simulink model "LFC_Fuzzy_AREA2"  (R2021a)
settings: Solver=VariableStepAuto  StartTime=0.0  StopTime=100  RelTol=1e-3
libraries: pid_lib x1, fuzblock x1, spspowerguiLib x1
settings Model: Creator=B.HARISH  LastModifiedBy=B.HARISH

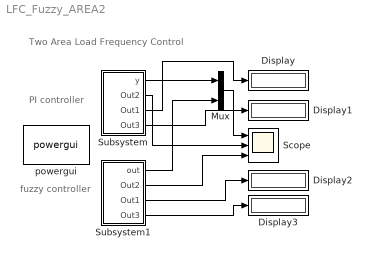
== system LFC_Fuzzy_AREA2 ==
  note: fuzzy controller
  note: PI controller
  note: Two Area Load Frequency Control
  Display{,1..3} (4 alike) : Display
  Mux : Mux  Inputs=2
  Scope : Scope  NumInputPorts=3
  Subsystem : Subsystem
  Subsystem1 : Subsystem
  powergui : spspowerguiLib/powergui  Priority=1  SimulationMode=Continuous  SampleTime=50e-6  frequency=60  Iterations=50  frequencyindice=60  Pbase=100e6  ErrMax=1e-4  UnitsV=kV  UnitsW=MW  buscounter=0  FunctionMessages=off  echomessages=off  EnableUseOfTLC=off  CurrentSourceSwitches=off  DisableSnubberDevices=off  DisableRonSwitches=off  DisableVfSwitches=off  DisplayEquations=off  AutomaticDiscreteSolvers=off  SolverType=Tustin/Backward Euler (TBE)  Interpol=off  ExternalGateDelay=off  methode=off  Ts=100  x0status=blocks  SPID=off  SwTol=0  HookPort=off  NonlinearTolerance=1e-4  nMaxIteration=100  ContinueOnMaxIteration=off  RestoreLinks=warning  ResistiveCurrentMeasurement=off  Frange=[0:2:500]  Ylog=off  Xlog=on  ShowGrid=off  save=off  variable=ZData  structure=0  ZoomFFT=off  StartTime=0.0  cycles=1  DisplayStyle=1  fundamental=60  FreqAxis=off  MaxFrequency=1000  frequencyindicesteady=1  RmsSteady=1  display=off
  wires:
  Subsystem1/2(Out2) -> Scope/3
  Subsystem/2(Out2) -> Scope/2
  Subsystem/1(y) -> Mux/1
  Subsystem1/1(out) -> Mux/2
  Mux/1 -> Scope/1
  Subsystem1/3(Out1) -> Display2/1
  Subsystem1/4(Out3) -> Display3/1
  Subsystem/3(Out1) -> Display/1
  Subsystem/4(Out3) -> Display1/1

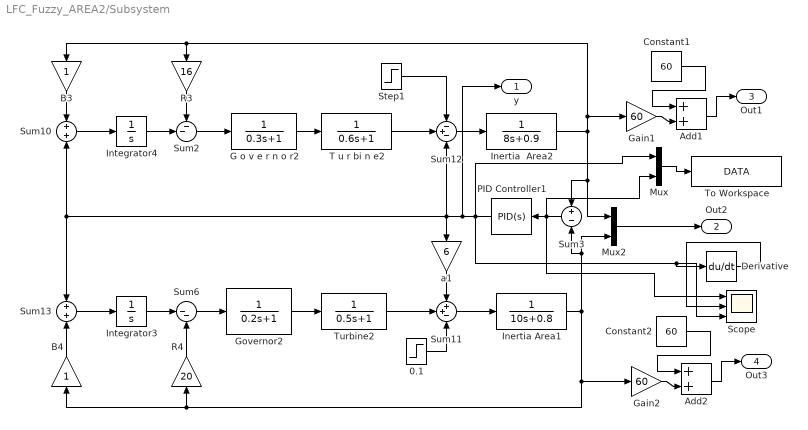
== system LFC_Fuzzy_AREA2/Subsystem ==
  0.1 : Step  Time=0  After=0.2  SampleTime=0
  Add1 : Sum
  Add2 : Sum
  B3 : Gain
  B4 : Gain
  Constant1 : Constant  Value=60
  Constant2 : Constant  Value=60
  Derivative : Derivative
  G o v e r n o r2 : TransferFcn  Denominator=[0.3 1]  ParameterTunability=Optimized
  Gain1 : Gain  Gain=60
  Gain2 : Gain  Gain=60
  Governor2 : TransferFcn  Denominator=[0.2 1]
  Inertia  Area2 : TransferFcn  Denominator=[8 0.9]
  Inertia Area1 : TransferFcn  Denominator=[10 0.8]
  Integrator3 : Integrator
  Integrator4 : Integrator
  Mux : Mux  Inputs=2
  Mux2 : Mux  Inputs=2
  PID Controller1 : pid_lib/PID Controller  Controller=PID  Form=Parallel  TimeDomain=Continuous-time  UseExternalTs=off  SampleTime=-1  IntegratorMethod=Forward Euler  FilterMethod=Forward Euler  ControllerParametersSource=internal  P=5.57550599969574  I=9.98117323449892  D=0.481439807722255  UseFilter=on  N=13.7016060269838  TunerSelectOption=Transfer Function Based (PID Tuner App)  InitialConditionSource=internal  InitialConditionForIntegrator=0  InitialConditionForFilter=0  DifferentiatorICPrevScaledInput=0  ExternalReset=none  TrackingMode=off  Kt=1  LimitOutput=off  SatLimitsSource=internal  UpperSaturationLimit=inf  LowerSaturationLimit=-inf  LinearizeAsGain=on  AntiWindupMode=none  Kb=1  POutMin=[]  POutMax=[]  IOutMin=[]  IOutMax=[]  DOutMin=[]  DOutMax=[]  NOutMin=[]  NOutMax=[]  SumOutMin=[]  SumOutMax=[]  SaturationOutMin=[]  SaturationOutMax=[]  PParamMin=[]  PParamMax=[]  IParamMin=[]  IParamMax=[]  DParamMin=[]  DParamMax=[]  NParamMin=[]  NParamMax=[]  KbParamMin=[]  KbParamMax=[]  KtParamMin=[]  KtParamMax=[]  KbOutMin=[]  KbOutMax=[]  KtOutMin=[]  KtOutMax=[]  IntegratorOutMin=[]  IntegratorOutMax=[]  FilterOutMin=[]  FilterOutMax=[]  SumI1OutMin=[]  SumI1OutMax=[]  SumI2OutMin=[]  SumI2OutMax=[]  SumI3OutMin=[]  SumI3OutMax=[]  SumI4OutMin=[]  SumI4OutMax=[]  SumDOutMin=[]  SumDOutMax=[]  DifferentiatorOutMin=[]  DifferentiatorOutMax=[]  FilterDiffOutCoefMin=[]  FilterDiffOutCoefMax=[]  ReciprocalOutMin=[]  ReciprocalOutMax=[]  SumDenOutMin=[]  SumDenOutMax=[]  SumNumOutMin=[]  SumNumOutMax=[]  DivideOutMin=[]  DivideOutMax=[]  UdiffTsProdOutMin=[]  UdiffTsProdOutMax=[]  NTsProdOutMin=[]  NTsProdOutMax=[]  UintegralTsProdOutMin=[]  UintegralTsProdOutMax=[]  UngainTsProdOutMin=[]  UngainTsProdOutMax=[]  IntegratorContinuousStateAttributes=''  IntegratorStateMustResolveToSignalObject=off  IntegratorRTWStateStorageClass=Auto  FilterContinuousStateAttributes=''  FilterStateMustResolveToSignalObject=off  FilterRTWStateStorageClass=Auto  ParallelPVariant=InternalParameters  IdealPVariant=Disabled  IVariant=InternalParameters  DVariant=InternalParameters  IntegratorVariant=Continuous  SatVariant=Disabled  AWVariant=Passthrough  PCopyVariant=Disabled  TRVariant=Disabled  FdbkBlocksVariant=Forward  IdealPFdbkVariant=Disabled  SatFdbkVariant=Disabled  DerivativeFilterVariant=ContFilter  NVariant=InternalParameters  NCopyVariant=Disabled  FilterICVariant=InternalICsFilter  IntegratorICVariant=InternalICs  ExternalResetVariant=Disabled  TRSumVariant=Passthrough  SumFdbkVariant=Disabled  SumVariant=Sum_PID  TsampFilterVariant=InternalTs  TsampNgainVariant=Passthrough  TsampIntegralVariant=Passthrough  ExternalSaturationOutDataTypeStr=Inherit: Same as second input
  R3 : Gain  Gain=16
  R4 : Gain  Gain=20
  Scope : Scope  NumInputPorts=3
  Step1 : Step  Time=0  After=0.2  SampleTime=0
  Sum10 : Sum
  Sum11 : Sum  Inputs=++-
  Sum12 : Sum  Inputs=-+-
  Sum13 : Sum
  Sum2 : Sum  Inputs=--|
  Sum3 : Sum  Inputs=+-
  Sum6 : Sum  Inputs=|--
  T u r bi n e2 : TransferFcn  Denominator=[0.6 1]
  To Workspace : ToWorkspace  VariableName=DATA  SaveFormat=Timeseries  SampleTime=-1
  Turbine2 : TransferFcn  Denominator=[0.5 1]
  a1 : Gain  Gain=6
  y : Outport
  Out2 : Outport  Port=2
  Out1 : Outport  Port=3
  Out3 : Outport  Port=4
  wires:
  PID Controller1/1 -> Derivative/1, Scope/3, y/1, a1/1, Sum13/1, Sum10/2, Sum12/3, Mux/1
  G o v e r n o r2/1 -> T u r bi n e2/1
  0.1/1 -> Sum11/3
  T u r bi n e2/1 -> Sum12/2
  a1/1 -> Sum11/1
  Inertia  Area2/1 -> Gain1/1, B3/1, R3/1, Mux2/1, Sum3/1
  Sum10/1 -> Integrator4/1
  Integrator3/1 -> Sum6/1
  R3/1 -> Sum2/1
  Sum11/1 -> Inertia Area1/1
  Sum13/1 -> Integrator3/1
  Sum6/1 -> Governor2/1
  Sum12/1 -> Inertia  Area2/1
  Turbine2/1 -> Sum11/2
  Governor2/1 -> Turbine2/1
  B4/1 -> Sum13/2
  Integrator4/1 -> Sum2/2
  B3/1 -> Sum10/1
  R4/1 -> Sum6/2
  Step1/1 -> Sum12/1
  Inertia Area1/1 -> Gain2/1, B4/1, R4/1, Sum3/2, Mux2/2
  Sum2/1 -> G o v e r n o r2/1
  Sum3/1 -> Scope/1, PID Controller1/1, Mux/2
  Mux2/1 -> Out2/1
  Mux/1 -> To Workspace/1
  Derivative/1 -> Scope/2
  Add1/1 -> Out1/1
  Constant1/1 -> Add1/1
  Gain1/1 -> Add1/2
  Add2/1 -> Out3/1
  Constant2/1 -> Add2/1
  Gain2/1 -> Add2/2

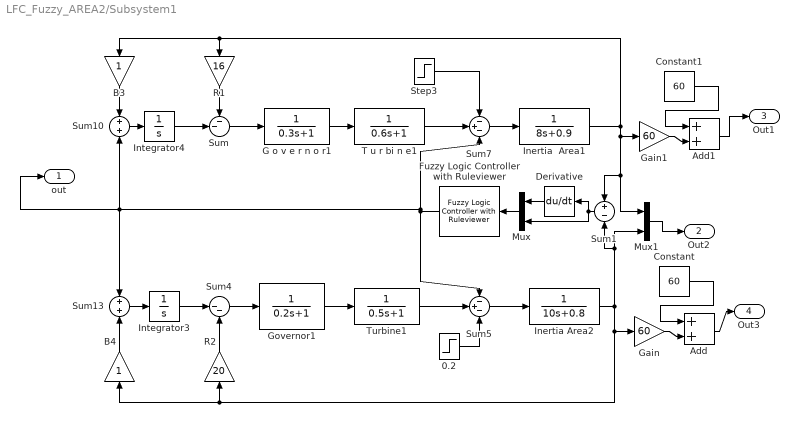
== system LFC_Fuzzy_AREA2/Subsystem1 ==
  0.2 : Step  Time=0  After=0.2  SampleTime=0
  Add : Sum
  Add1 : Sum
  B3 : Gain
  B4 : Gain
  Constant : Constant  Value=60
  Constant1 : Constant  Value=60
  Derivative : Derivative
  Fuzzy Logic Controller with Ruleviewer : fuzblock/Fuzzy Logic  Controller  with Ruleviewer  fismatrix=LFC_A2  Ts=2
  G o v e r n o r1 : TransferFcn  Denominator=[0.3 1]  ParameterTunability=Optimized
  Gain : Gain  Gain=60
  Gain1 : Gain  Gain=60
  Governor1 : TransferFcn  Denominator=[0.2 1]
  Inertia  Area1 : TransferFcn  Denominator=[8 0.9]
  Inertia Area2 : TransferFcn  Denominator=[10 0.8]
  Integrator3 : Integrator
  Integrator4 : Integrator
  Mux : Mux  Inputs=2
  Mux1 : Mux  Inputs=2
  R1 : Gain  Gain=16
  R2 : Gain  Gain=20
  Step3 : Step  Time=0  After=0.2  SampleTime=0
  Sum : Sum  Inputs=--|
  Sum1 : Sum  Inputs=+-
  Sum10 : Sum
  Sum13 : Sum
  Sum4 : Sum  Inputs=|--
  Sum5 : Sum  Inputs=-+-
  Sum7 : Sum  Inputs=-+-
  T u r bi n e1 : TransferFcn  Denominator=[0.6 1]
  Turbine1 : TransferFcn  Denominator=[0.5 1]
  out : Outport
  Out2 : Outport  Port=2
  Out1 : Outport  Port=3
  Out3 : Outport  Port=4
  wires:
  Inertia Area2/1 -> Gain/1, B4/1, R2/1, Sum1/2, Mux1/2
  Sum7/1 -> Inertia  Area1/1
  Inertia  Area1/1 -> Mux1/1, Sum1/1, Gain1/1, B3/1, R1/1
  R1/1 -> Sum/1
  R2/1 -> Sum4/2
  Turbine1/1 -> Sum5/2
  Governor1/1 -> Turbine1/1
  G o v e r n o r1/1 -> T u r bi n e1/1
  Sum4/1 -> Governor1/1
  Mux1/1 -> Out2/1
  Sum/1 -> G o v e r n o r1/1
  Fuzzy Logic Controller with Ruleviewer/1 -> out/1, Sum13/1, Sum10/2, Sum7/3, Sum5/1
  Sum5/1 -> Inertia Area2/1
  T u r bi n e1/1 -> Sum7/2
  Step3/1 -> Sum7/1
  0.2/1 -> Sum5/3
  Sum1/1 -> Mux/2, Derivative/1
  Sum10/1 -> Integrator4/1
  Sum13/1 -> Integrator3/1
  B4/1 -> Sum13/2
  B3/1 -> Sum10/1
  Integrator4/1 -> Sum/2
  Integrator3/1 -> Sum4/1
  Mux/1 -> Fuzzy Logic Controller with Ruleviewer/1
  Derivative/1 -> Mux/1
  Constant/1 -> Add/1
  Gain/1 -> Add/2
  Add/1 -> Out3/1
  Add1/1 -> Out1/1
  Gain1/1 -> Add1/2
  Constant1/1 -> Add1/1
